simulink model "Simple_Asynchronous"  (R2016a)
settings: Solver=ode45  StartTime=0.0  StopTime=40  RelTol=1e-3
libraries: powerlib x16
settings Model: Creator=lm  LastModifiedBy=Jasonkay
settings DataIOCC: LimitDataPoints=on  SaveFormat=Array  SignalLoggingSaveFormat=ModelDataLogs
settings OptimizationCC: ExpressionDepthLimit=2147483647
settings DebuggingCC: UnderspecifiedInitializationDetection=Classic  MergeDetectMultiDrivingBlocksExec=none  SolverPrmCheckMsg=warning  FcnCallInpInsideContextMsg=UseLocalSettings  StateNameClashWarn=warning
settings HardwareCC: ProdBitPerPointer=32  ProdLargestAtomicFloat=None  ProdIntDivRoundTo=Undefined  ProdEndianess=Unspecified  ProdWordSize=32  ProdHWDeviceType=32-bit Generic
settings ModelReferenceCC: PropagateSignalLabelsOutOfModel=off
settings GRTTargetCC: CombineOutputUpdateFcns=off  GRTInterface=on
settings ConfigComp: CovModelRefEnable=Off

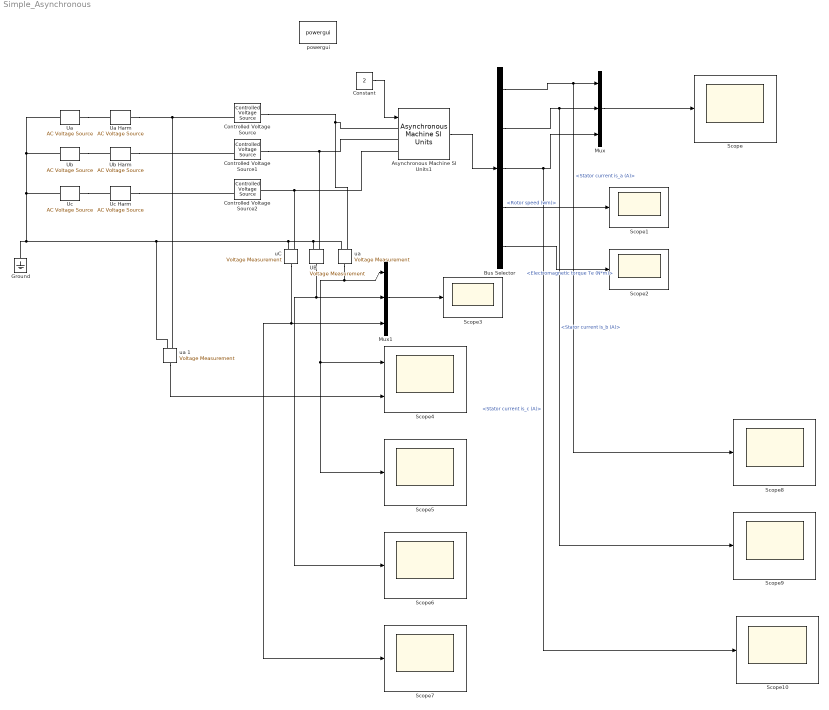
== system Simple_Asynchronous ==
  Asynchronous Machine SI Units1 : powerlib/Machines/Asynchronous Machine SI Units  RotorType=Squirrel-cage  PresetModel="17:  20 HP (15KW)   400 V 50Hz 1460 RPM"  MechanicalLoad=Torque Tm  ShowDetailedParameters=on  ReferenceFrame=Rotor  Units=SI  MeasurementBus=off  NominalParameters=[1.5e+04 400 50]  Stator=[0.2147 0.000991]  Rotor=[0.2205 0.000991]  Cage1=[0.4155 0.002066]  Cage2=[0.4168 0.0003495]  Lm=0.06419  Mechanical=[0.102 0.009541 2]  PolePairs=2  InitialConditions=[0 0 0 0 0 0 0 0]  SimulateSaturation=off  Saturation=[14.03593122, 27.81365428, 53.79336849, 72.68890987, 97.98006896, 148.6815601, 215.7428561, 302.9841135, 428.7778367 ; 230, 322, 414, 460, 506, 552, 598, 644, 690]  LoadFlowParameters=1492000  TsPowergui=0  TsBlock=-1  IterativeModel=Trapezoidal non iterative  IterativeDiscreteModel=Trapezoidal non iterative  Pmec=1.492e+006
  Bus Selector : BusSelector  OutputSignals=Stator measurements.Stator current is_a (A),Stator measurements.Stator current is_b (A),Stator measurements.Stator current is_c (A),Mechanical.Rotor speed (wm),Mechanical.Electromagnetic torque Te (N*m)
  Constant : Constant  Value=2
  Controlled Voltage Source : powerlib/Electrical Sources/Controlled Voltage Source  Initialize=on  Source_Type=AC  Amplitude=0  Phase=0  Frequency=0  Measurements=None
  Controlled Voltage Source1 : powerlib/Electrical Sources/Controlled Voltage Source  Initialize=on  Source_Type=AC  Amplitude=0  Phase=0  Frequency=0  Measurements=None
  Controlled Voltage Source2 : powerlib/Electrical Sources/Controlled Voltage Source  Initialize=on  Source_Type=AC  Amplitude=0  Phase=0  Frequency=0  Measurements=None
  Ground : powerlib/Elements/Ground  LConnTagsString=a
  Mux : Mux  Inputs=3
  Mux1 : Mux  Inputs=3
  Scope{,1..3,5..10} (10 alike) : Scope
  Scope4 : Scope  NumInputPorts=2
  "UB " : powerlib/Measurements/Voltage Measurement  PhasorSimulation=off  OutputType=Complex  PSBequivalent=0
  "Ua " : powerlib/Electrical Sources/AC Voltage Source  Amplitude=220 * sqrt(2)  Phase=0  Frequency=50  SampleTime=0  Measurements=None  BusType=swing  Pref=10e3  Qref=0  Qmin=-inf  Qmax=+inf
  Ua Harm : powerlib/Electrical Sources/AC Voltage Source  Amplitude=15 * sqrt(2)  Phase=0  Frequency=50.5  SampleTime=0  Measurements=None  BusType=swing  Pref=10e3  Qref=0  Qmin=-inf  Qmax=+inf
  "Ub " : powerlib/Electrical Sources/AC Voltage Source  Amplitude=220 * sqrt(2)  Phase=240  Frequency=50  SampleTime=0  Measurements=None  BusType=swing  Pref=10e3  Qref=0  Qmin=-inf  Qmax=+inf
  Ub Harm : powerlib/Electrical Sources/AC Voltage Source  Amplitude=15 * sqrt(2)  Phase=240  Frequency=50.5  SampleTime=0  Measurements=None  BusType=swing  Pref=10e3  Qref=0  Qmin=-inf  Qmax=+inf
  "Uc " : powerlib/Electrical Sources/AC Voltage Source  Amplitude=220 * sqrt(2)  Phase=120  Frequency=50  SampleTime=0  Measurements=None  BusType=swing  Pref=10e3  Qref=0  Qmin=-inf  Qmax=+inf
  Uc Harm : powerlib/Electrical Sources/AC Voltage Source  Amplitude=15 * sqrt(2)  Phase=120  Frequency=50.5  SampleTime=0  Measurements=None  BusType=swing  Pref=10e3  Qref=0  Qmin=-inf  Qmax=+inf
  powergui : powerlib/powergui  Priority=1  SimulationMode=Discrete  SolverType=Tustin/Backward Euler (TBE)  SampleTime=1 / (160 * 50)  frequency=60  SPID=off  DisableSnubberDevices=off  DisableRonSwitches=off  DisableVfSwitches=off  SwTol=0  DisplayEquations=off  Interpol=off  ExternalGateDelay=off  methode=off  Ts=10  FunctionMessages=off  echomessages=off  HookPort=off  EnableUseOfTLC=off  x0status=blocks  frequencyindice=50  Pbase=100e6  ErrMax=1e-4  Iterations=50  UnitsV=kV  UnitsW=MW  buscounter=0  RestoreLinks=warning  ResistiveCurrentMeasurement=off  Frange=[0:2:500]  Ylog=off  Xlog=on  ShowGrid=off  save=off  variable=ZData  structure=Ua1  ZoomFFT=off  StartTime=0.5  cycles=100  DisplayStyle=2  fundamental=50  FreqAxis=off  MaxFrequency=100  frequencyindicesteady=1  RmsSteady=1  display=off
  "uC " : powerlib/Measurements/Voltage Measurement  PhasorSimulation=off  OutputType=Complex  PSBequivalent=0
  "ua " : powerlib/Measurements/Voltage Measurement  PhasorSimulation=off  OutputType=Complex  PSBequivalent=0
  ua 1 : powerlib/Measurements/Voltage Measurement  PhasorSimulation=off  OutputType=Complex  PSBequivalent=0
  wires:
  Asynchronous Machine SI Units1/1 -> Bus Selector/1
  Bus Selector/1 -> Scope8/1, Mux/1  "<Stator current is_a (A)>"
  Bus Selector/2 -> Scope9/1, Mux/2  "<Stator current is_b (A)>"
  Bus Selector/3 -> Scope10/1, Mux/3  "<Stator current is_c (A)>"
  Mux/1 -> Scope/1
  Bus Selector/4 -> Scope1/1  "<Rotor speed (wm)>"
  Bus Selector/5 -> Scope2/1  "<Electromagnetic torque Te (N*m)>"
  Constant/1 -> Asynchronous Machine SI Units1/1
  "ua "/1 -> Scope5/1, Scope4/1, Mux1/1
  "UB "/1 -> Scope6/1, Mux1/2
  "uC "/1 -> Mux1/3, Scope7/1
  ua 1/1 -> Scope4/2
  Mux1/1 -> Scope3/1
  connections:
  "ua "/LConn2 -- "UB "/LConn2 -- "uC "/LConn2 -- ua 1/LConn2 -- Ground/LConn1 -- "Ua "/LConn1 -- "Ub "/LConn1 -- "Uc "/LConn1
  Asynchronous Machine SI Units1/LConn2 -- "UB "/LConn1 -- Controlled Voltage Source1/RConn1
  Asynchronous Machine SI Units1/LConn1 -- Controlled Voltage Source/RConn1 -- "ua "/LConn1
  Controlled Voltage Source/LConn1 -- Ua Harm/RConn1 -- ua 1/LConn1
  "Ub "/RConn1 -- Ub Harm/LConn1
  "Uc "/RConn1 -- Uc Harm/LConn1
  "uC "/LConn1 -- Controlled Voltage Source2/RConn1 -- Asynchronous Machine SI Units1/LConn3
  "Ua "/RConn1 -- Ua Harm/LConn1
  Ub Harm/RConn1 -- Controlled Voltage Source1/LConn1
  Uc Harm/RConn1 -- Controlled Voltage Source2/LConn1
